simulink model "Ex4_1_sim"  (R2014a)
settings: Solver=ode45  StartTime=0.0  StopTime=Endtime  RelTol=1e-3
values from neighbouring files (symbols this model uses):
  d0 = 25.0    (= 25)    [Ex4_1.m]
  K = 1.15    [Ex4_1.m]
  L = 15    [Ex4_1.m]
  T = 1115    [Ex4_1.m]
settings Model: Creator=Shin  LastModifiedBy=Shin
settings OptimizationCC: SimCompilerOptimization=off
settings DebuggingCC: MergeDetectMultiDrivingBlocksExec=error  FrameProcessingCompatibilityMsg=error
settings RTWCC: RTWCompilerOptimization=off

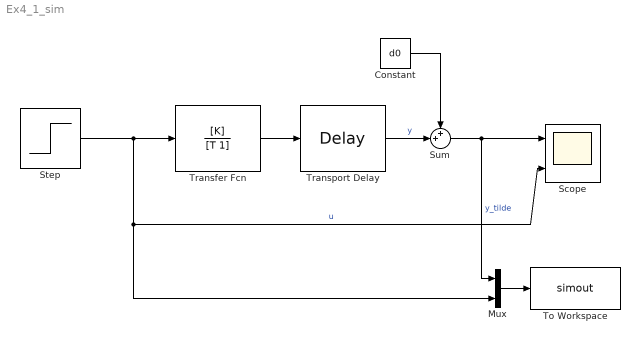
== system Ex4_1_sim ==
  Constant : Constant  Value=d0
  Mux : Mux  Inputs=2
  Scope : Scope  NumInputPorts=2
      settings: YMin=25~0  YMax=65~350
  Step : Step  Time=5  After=u  SampleTime=0
  Sum : Sum  Inputs=++|
  To Workspace : ToWorkspace  VariableName=simout  SaveFormat=Timeseries  SampleTime=-1
  Transfer Fcn : TransferFcn  Numerator=[K]  Denominator=[T 1]
  Transport Delay : TransportDelay  DelayTime=L
  wires:
  Transfer Fcn/1 -> Transport Delay/1
  Constant/1 -> Sum/1
  Transport Delay/1 -> Sum/2  "y"
  Sum/1 -> Scope/1, Mux/1  "y_tilde"
  Step/1 -> Mux/2, Scope/2, Transfer Fcn/1  "u"
  Mux/1 -> To Workspace/1
